simulink model "DesignSplineSplitter"  (R2016b)
settings: Solver=VariableStepAuto  StartTime=0.0  StopTime=10.0  RelTol=1e-3
settings Model: DataDictionary=DataDictionary.sldd  Creator=Taeke  LastModifiedBy=Taeke

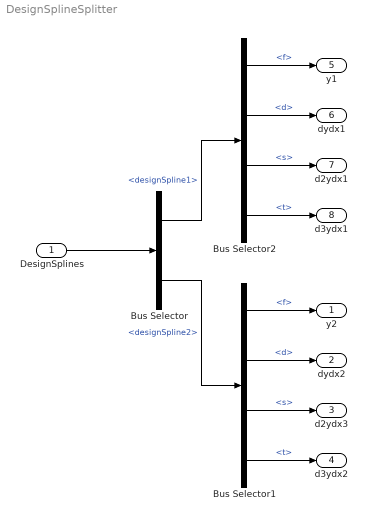
== system DesignSplineSplitter ==
  DesignSplines : Inport  OutDataTypeStr=Bus: designSplineTotal
  Bus Selector : BusSelector  OutputSignals=designSpline1,designSpline2
  Bus Selector1 : BusSelector  OutputSignals=f,d,s,t
  Bus Selector2 : BusSelector  OutputSignals=f,d,s,t
  y2 : Outport
  dydx2 : Outport  Port=2
  d2ydx3 : Outport  Port=3
  d3ydx2 : Outport  Port=4
  y1 : Outport  Port=5
  dydx1 : Outport  Port=6
  d2ydx1 : Outport  Port=7
  d3ydx1 : Outport  Port=8
  wires:
  DesignSplines/1 -> Bus Selector/1
  Bus Selector/2 -> Bus Selector1/1  "<designSpline2>"
  Bus Selector/1 -> Bus Selector2/1  "<designSpline1>"
  Bus Selector2/1 -> y1/1  "<f>"
  Bus Selector2/2 -> dydx1/1  "<d>"
  Bus Selector2/3 -> d2ydx1/1  "<s>"
  Bus Selector2/4 -> d3ydx1/1  "<t>"
  Bus Selector1/1 -> y2/1  "<f>"
  Bus Selector1/2 -> dydx2/1  "<d>"
  Bus Selector1/3 -> d2ydx3/1  "<s>"
  Bus Selector1/4 -> d3ydx2/1  "<t>"
